simulink model "controller_frequency_check_2021"  (R2021b)
settings: Solver=VariableStepAuto  StartTime=0.0  StopTime=50  RelTol=1e-3
values from neighbouring files (symbols this model uses):
  A = [0,  0,                             1,                           0 ... (first row only)    [main.m]    (also in taak.m = [0, 0, 1, 0; 0, 0, 0, 1; 0, K_stiff/J_h, -((K_g)^2*K_m*K_b)/)
  B = [ 0 ... (first row only)    [main.m]    (also in taak.m = [0; 0; (K_m*K_g)/(R_m*J_h);-(K_m*K_g)/(R_m*J_h)])
  C = [1 0 0 0 ... (first row only)    [main.m]
undefined symbols (not defined in the file or in its folder): K
libraries: simulink x1
settings Model: Creator=Sofie  LastModifiedBy=Sofie
settings DebuggingCC: UnconnectedInputMsg=none  UnconnectedOutputMsg=none  UnconnectedLineMsg=none
settings ModelReferenceCC: EnableRefExpFcnMdlSchedulingChecks=off
settings RTWCC: DLArmComputeVersion=20.02.1

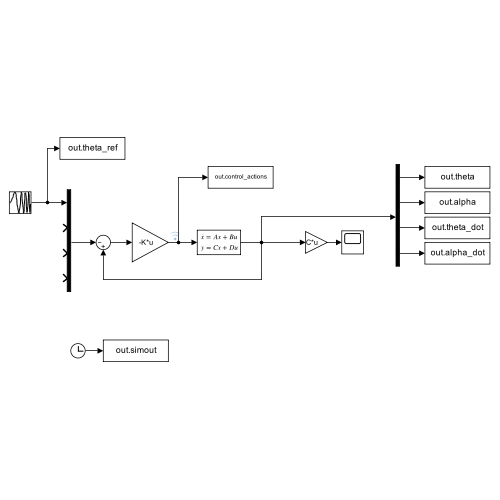
[thumbnail: Simulink's stored preview of the top-level diagram]
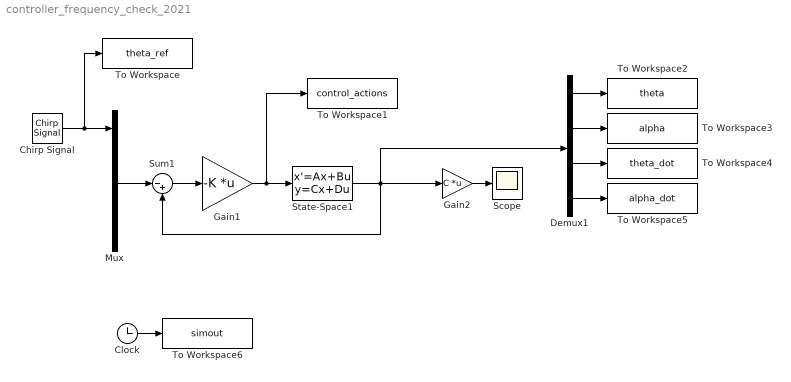
== system controller_frequency_check_2021 ==
  Chirp Signal : simulink/Sources/Chirp Signal  f1=0  T=50  f2=100
  Clock : Clock
  Demux1 : Demux
  Gain1 : Gain  Gain=-K  Multiplication=Matrix(K*u)
  Gain2 : Gain  Gain=C  Multiplication=Matrix(K*u)
  Mux : Mux
  Scope : Scope
  State-Space1 : StateSpace  A=A  B=B  C=eye(4)  D=zeros(4,1)  InitialCondition=[0,0,0,0]
  Sum1 : Sum  Inputs=|-+
  To Workspace : ToWorkspace  VariableName=theta_ref  SaveFormat=Timeseries  SampleTime=-1
  To Workspace1 : ToWorkspace  VariableName=control_actions  SaveFormat=Timeseries  SampleTime=-1
  To Workspace2 : ToWorkspace  VariableName=theta  SaveFormat=Timeseries  SampleTime=-1
  To Workspace3 : ToWorkspace  VariableName=alpha  SaveFormat=Timeseries  SampleTime=-1
  To Workspace4 : ToWorkspace  VariableName=theta_dot  SaveFormat=Timeseries  SampleTime=-1
  To Workspace5 : ToWorkspace  VariableName=alpha_dot  SaveFormat=Timeseries  SampleTime=-1
  To Workspace6 : ToWorkspace  VariableName=simout  SaveFormat=Timeseries  SampleTime=-1
  wires:
  Mux/1 -> Sum1/1
  Demux1/3 -> To Workspace4/1
  Demux1/4 -> To Workspace5/1
  Sum1/1 -> Gain1/1
  Demux1/1 -> To Workspace2/1
  State-Space1/1 -> Sum1/2, Demux1/1, Gain2/1
  Chirp Signal/1 -> To Workspace/1, Mux/1
  Gain1/1 -> To Workspace1/1, State-Space1/1
  Demux1/2 -> To Workspace3/1
  Gain2/1 -> Scope/1
  Clock/1 -> To Workspace6/1
